simulink model "prediction"  (R2012b)
settings: Solver=FixedStepDiscrete  StartTime=0.0  StopTime=inf  MaxStep=0.0001  RelTol=1e-3
libraries: MAVLink_Block x1
settings Model: Creator=fede  LastModifiedBy=fede

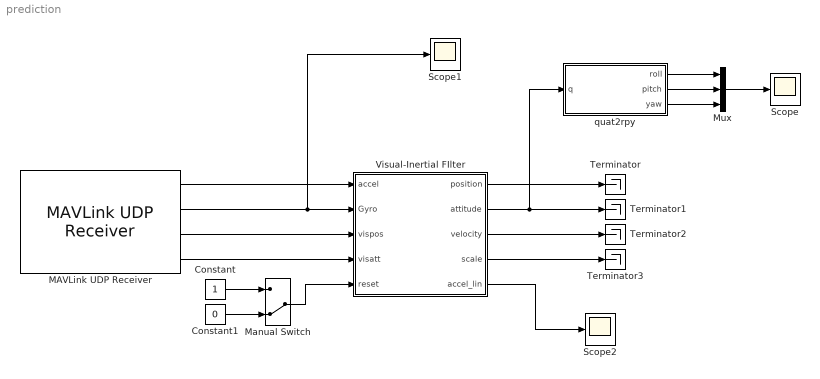
== system prediction ==
  Constant : Constant
  Constant1 : Constant  Value=0
  MAVLink UDP Receiver : MAVLink_Block/MAVLink UDP Receiver  Priority=1  Port=14550  FS=0.001  accel=on  gyro=on  magn=off  vispos=on  visatt=on  msg_vector=0
  Manual Switch : ManualSwitch  CurrentSetting=0
  Mux : Mux  Inputs=3
  Scope : Scope
      settings: TimeRange=250  YMin=-0.375  YMax=0.15
  Scope1 : Scope
      settings: TimeRange=250  YMin=-0.375  YMax=0.15
  Scope2 : Scope
      settings: TimeRange=250  YMin=-6  YMax=10  SaveName=ScopeData2
  Terminator{,1..3} (4 alike) : Terminator
  Visual-Inertial FIlter : Subsystem  TreatAsAtomicUnit=on
  quat2rpy : MATLAB Function  TreatAsAtomicUnit=on
  wires:
  MAVLink UDP Receiver/4 -> Visual-Inertial FIlter/4(visatt)
  MAVLink UDP Receiver/2 -> Scope1/1, Visual-Inertial FIlter/2(Gyro)
  MAVLink UDP Receiver/1 -> Visual-Inertial FIlter/1(accel)
  MAVLink UDP Receiver/3 -> Visual-Inertial FIlter/3(vispos)
  Visual-Inertial FIlter/4(scale) -> Terminator3/1
  Visual-Inertial FIlter/3(velocity) -> Terminator2/1
  Visual-Inertial FIlter/2(attitude) -> quat2rpy/1(q), Terminator1/1
  Visual-Inertial FIlter/1(position) -> Terminator/1
  Manual Switch/1 -> Visual-Inertial FIlter/5(reset)
  Constant/1 -> Manual Switch/1
  Constant1/1 -> Manual Switch/2
  quat2rpy/2(pitch) -> Mux/2
  quat2rpy/1(roll) -> Mux/1
  quat2rpy/3(yaw) -> Mux/3
  Mux/1 -> Scope/1
  Visual-Inertial FIlter/5(accel_lin) -> Scope2/1

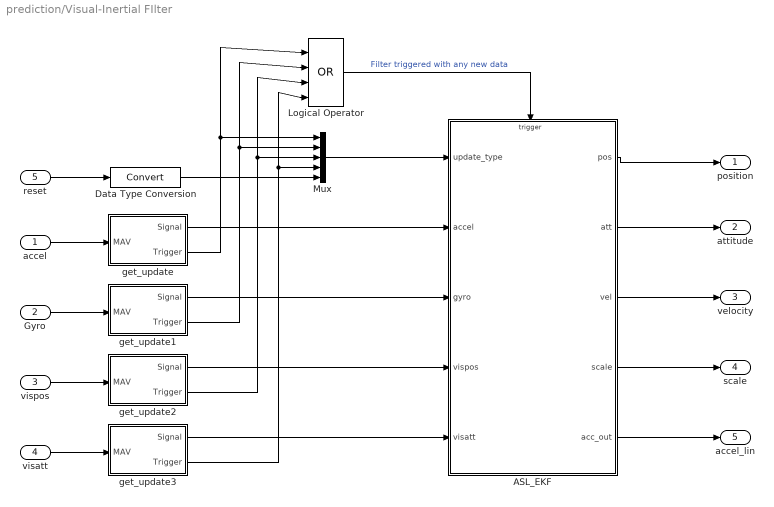
== system prediction/Visual-Inertial FIlter ==
  accel : Inport
  Gyro : Inport  Port=2
  vispos : Inport  Port=3
  visatt : Inport  Port=4
  reset : Inport  Port=5
  ASL_EKF : MATLAB Function  TreatAsAtomicUnit=on
  Data Type Conversion : DataTypeConversion
  Logical Operator : Logic  Operator=OR  Inputs=4  IconShape=distinctive  AllPortsSameDT=off  OutDataTypeStr=boolean
  Mux : Mux  Inputs=5
  get_update : Subsystem
  get_update1 : Subsystem
  get_update2 : Subsystem
  get_update3 : Subsystem
  position : Outport
  attitude : Outport  Port=2
  velocity : Outport  Port=3
  scale : Outport  Port=4
  accel_lin : Outport  Port=5
  wires:
  ASL_EKF/1(pos) -> position/1
  ASL_EKF/2(att) -> attitude/1
  ASL_EKF/3(vel) -> velocity/1
  ASL_EKF/4(scale) -> scale/1
  accel/1 -> get_update/1(MAV)
  visatt/1 -> get_update3/1(MAV)
  vispos/1 -> get_update2/1(MAV)
  Gyro/1 -> get_update1/1(MAV)
  get_update/2(Trigger) -> Logical Operator/1, Mux/1
  get_update1/2(Trigger) -> Logical Operator/2, Mux/2
  get_update2/2(Trigger) -> Logical Operator/3, Mux/3
  Logical Operator/1 -> ASL_EKF/Trigger  "Filter triggered with any new data"
  get_update/1(Signal) -> ASL_EKF/2(accel)
  get_update1/1(Signal) -> ASL_EKF/3(gyro)
  get_update3/2(Trigger) -> Logical Operator/4, Mux/4
  Mux/1 -> ASL_EKF/1(update_type)
  get_update2/1(Signal) -> ASL_EKF/4(vispos)
  get_update3/1(Signal) -> ASL_EKF/5(visatt)
  reset/1 -> Data Type Conversion/1
  Data Type Conversion/1 -> Mux/5
  ASL_EKF/5(acc_out) -> accel_lin/1

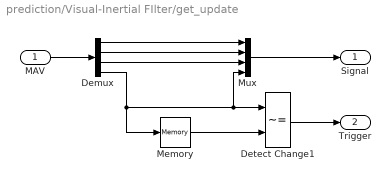
== system prediction/Visual-Inertial FIlter/get_update ==
  MAV : Inport
  Demux : Demux
  Detect Change1 : RelationalOperator  Operator=~=  OutDataTypeStr=boolean
  Memory : Memory
  Mux : Mux
  Signal : Outport
  Trigger : Outport  Port=2
  wires:
  Demux/4 -> Mux/4, Detect Change1/1, Memory/1
  Memory/1 -> Detect Change1/2
  Demux/3 -> Mux/3
  Demux/2 -> Mux/2
  Mux/1 -> Signal/1
  MAV/1 -> Demux/1
  Demux/1 -> Mux/1
  Detect Change1/1 -> Trigger/1

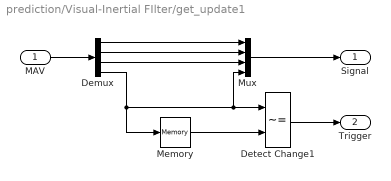
== system prediction/Visual-Inertial FIlter/get_update1 ==
  MAV : Inport
  Demux : Demux
  Detect Change1 : RelationalOperator  Operator=~=  OutDataTypeStr=boolean
  Memory : Memory
  Mux : Mux
  Signal : Outport
  Trigger : Outport  Port=2
  wires:
  Demux/1 -> Mux/1
  MAV/1 -> Demux/1
  Mux/1 -> Signal/1
  Detect Change1/1 -> Trigger/1
  Demux/2 -> Mux/2
  Demux/3 -> Mux/3
  Memory/1 -> Detect Change1/2
  Demux/4 -> Memory/1, Detect Change1/1, Mux/4

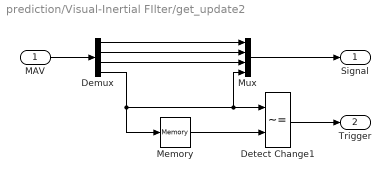
== system prediction/Visual-Inertial FIlter/get_update2 ==
  MAV : Inport
  Demux : Demux
  Detect Change1 : RelationalOperator  Operator=~=  OutDataTypeStr=boolean
  Memory : Memory
  Mux : Mux
  Signal : Outport
  Trigger : Outport  Port=2
  wires:
  Demux/4 -> Mux/4, Detect Change1/1, Memory/1
  Memory/1 -> Detect Change1/2
  Demux/3 -> Mux/3
  Demux/2 -> Mux/2
  Detect Change1/1 -> Trigger/1
  Mux/1 -> Signal/1
  MAV/1 -> Demux/1
  Demux/1 -> Mux/1

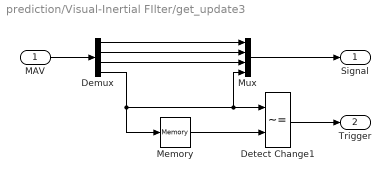
== system prediction/Visual-Inertial FIlter/get_update3 ==
  MAV : Inport
  Demux : Demux
  Detect Change1 : RelationalOperator  Operator=~=  OutDataTypeStr=boolean
  Memory : Memory
  Mux : Mux
  Signal : Outport
  Trigger : Outport  Port=2
  wires:
  Demux/1 -> Mux/1
  MAV/1 -> Demux/1
  Mux/1 -> Signal/1
  Detect Change1/1 -> Trigger/1
  Demux/2 -> Mux/2
  Demux/3 -> Mux/3
  Memory/1 -> Detect Change1/2
  Demux/4 -> Memory/1, Detect Change1/1, Mux/4

== matlab function prediction/Visual-Inertial FIlter/ASL_EKF ==
  data: update_type input; pos output; att output; vel output; accel input; gyro input; vispos input; visatt input; scale output; acc_out output
  events: anyData input RISING_EDGE_EVENT
function [pos, att, vel, scale, acc_out] = full_filter(update_type, accel, gyro, vispos, visatt)
%#codegen

% - Filter implementation from:
% S. Weiss and R. Siegwart, “Real-time metric state estimation for modular 
% vision-inertial systems,” in Robotics and Automation (ICRA), 2011 IEEE 
% International Conference on, 2011, pp. 4531–4537.


    persistent state old_state att_init
    
    % It is defined that the callback from the IMU will be at the
    % accelerometer rate. This is means we will downsample gyro by a factor
    % of 2: 100Hz
    
    
    
    type = 0;
    reset = false;
    if update_type(1) && ~update_type(3)
        type = 1;
    end
    if ~update_type(1) && update_type(3)
        type = 2;
    end
    if update_type(1) && update_type(3)
        type = 3;
    end
    
    if update_type(5)
        reset = true;
    end
    
    if isempty(state) || reset
        att_init = false;
        state.accel_l = zeros(3,1);
        state.pos = zeros(3,1);
        state.vel = zeros(3,1);
        state.att = zeros(4,1);
        state.scale = 0.1;
        state.b_gyro = zeros(3,1);
        state.b_accel = zeros(3,1);
        % calibration states ... keep constant!
        state.cam2imu_rot = zeros(4,1); 
        state.cam2imu_dist = zeros(3,1);
        
    end
    
    % Fill structures
    IMU.gyro = gyro(1:3);
    IMU.accel = accel(1:3);
    IMU.T = accel(end);
    
    vision.vispos = vispos(1:3);
    vision.visatt = visatt(1:3);
    vision.T = vispos(end);
    
    state.IMU = IMU;
    state.vision = vision;
    
    if isempty(old_state)
        pos = state.pos;
        vel = state.vel;
        att = state.att;
        scale = state.scale;
        acc_out = state.accel_l;
        old_state = state;
        return;
    end
    
    switch type
        case 0
%             disp('No update');
            
        case 1 % IMU callback only when accelerometer
            if att_init
                state = IMU_callback(state, old_state);
            else
                [state, att_init] = init_attitude(state, reset);
            end
            
        case 2 % Vision callback
            disp('vision callback');
        
        case 3 % Vision and IMU callback
            disp('vision and imu callback');      
    end

    % - Select output signals.
    pos = state.pos;
    vel = state.vel;
    att = state.att;
    scale = state.scale;
    acc_out = state.accel_l;
    old_state = state;
end


% ----------------------------------------------------------------------- %

% Here we will define functions to be called for each update type, given
% the sate as an argument and returning such state with its update or
% preditcion. 

function state_out = IMU_callback(state, state_old)
    dt = state.IMU.T - state_old.IMU.T;

    ew = state.IMU.gyro;
    ewold = state_old.IMU.gyro;
    ea = state.IMU.accel;
    eaold = state_old.IMU.accel;
    
    omega = omegaJPL(ew);
    omegaOld = omegaJPL(ewold);
    omegaMean = omegaJPL( (ew + ewold)./2 );
    
    state.att = (eye(4) + 0.5*omega*dt)*state_old.att;
    state.att = bsxfun(@rdivide, state.att, sqrt(sum(state.att.^2)));
    
    dv = ( quaternion(state.att)*ea + quaternion(state.att)*eaold ) ./ 2;
    dv = dv + [0 0 9.81]';
    state.vel = state_old.vel + dv*dt;
    state.pos = state_old.pos + (state.vel + state_old.vel)./2*dt;
    state.accel_l = dv;
    state_out = state;
end

function [state_out, att_init] = init_attitude(state, reset)
    % Assume the phone is still.
    % Extract the initial attitude from the accelerometer reading.
    
    persistent count_samples acum_acc
    
    if isempty(count_samples) || reset
        count_samples = 0;
    end
    
    if isempty(acum_acc) || reset
        acum_acc = zeros(3,100);    
    end
    
    if count_samples < 100
        count_samples = count_samples + 1;
        acum_acc(:,count_samples) = state.IMU.accel;
        state_out = state;
        att_init = false;
    else
        % Get attitude
        acc = mean(acum_acc, 2);
        acc = bsxfun(@rdivide, acc, sqrt(sum(acc.^2)));  
        disp('mean acceleration is')
        disp(acc);
        
        % get the quaternion between the direction of gravity and the
        % desired alignment axis, the z-axis.
% (http://www.euclideanspace.com/maths/algebra/vectors/angleBetween/index.htm)
        n = cross(acc, [0 0 -1]');
        d = dot(acc, [0 0 -1]');
        q = [n;d+1];
        q = bsxfun(@rdivide, q, sqrt(sum(q.^2)));  
        state_out = state;
        state_out.att = q;
        att_init = true;
    end 
end

== matlab function prediction/quat2rpy ==
  data: q input; roll output; pitch output; yaw output
function [roll, pitch, yaw] = quat2rpy( q )
%#codegen
    qx = q(1);
    qy = q(2);
    qz = q(3);
    qw = q(4);

    roll = atan2(2*qy*qw-2*qx*qz , 1 - 2*qy^2 - 2*qz^2);
    pitch = asin(2*qx*qy + 2*qz*qw);
    yaw = atan2(2*qx*qw-2*qy*qz , 1 - 2*qx^2 - 2*qz^2);
end
